simulink model "SPEED_CALCULATOIN"  (R2024b)
settings: Solver=FixedStepDiscrete  StartTime=0.0  StopTime=10.0  FixedStep=0.001  RelTol=1e-3
undefined symbols (not defined in the file): CONST_10000_u32, CONST_ONE_u8, DEFAULT_MAX_SPD_LIM_u16, DEFAULT_PAS_SPD_U16, DEFAULT_SPD_LIM_U16, ECO_MODE_SPD_LIM_u16, FITNESS_MODE_U8, MAX_SPD_VALUE_U16, MIN_SPD_VALUE_U16, PAS_FIVE_SPD_THSD_U16, PAS_FOUR_SPD_THSD_U16, PAS_ONE_SPD_THSD_U16, PAS_THREE_SPD_THSD_U16, PAS_TWO_SPD_THSD_U16, RPM_TO_KMPH_CONST_u32, SPD_BUFFER_u16, SPD_CONV_METER_u16, THROTTLE_SPD_LIM_U16, THROTTLE_THRESHOLD_U16, URBAN_MODE_SPD_LIM_u16, WALKMODE_SPD_LIM_U16
libraries: simulink x3
settings Model: DataDictionary=MCU_FOC_MAIN_DD.sldd  Creator=415  LastModifiedBy=415
settings OptimizationCC: DefaultParameterBehavior=Inlined  UseDivisionForNetSlopeComputation=on  GainParamInheritBuiltInType=on  UseFloatMulNetSlope=on  UseSpecifiedMinMax=on  InlineInvariantSignals=on  BitwiseOrLogicalOp=Bitwise operator  PassReuseOutputArgsAs=Individual arguments  ZeroExternalMemoryAtStartup=off  ZeroInternalMemoryAtStartup=off  NoFixptDivByZeroProtection=on  EfficientFloat2IntCast=on  LifeSpan=inf  OptimizeBlockOrder=speed  DifferentSizesBufferReuse=on  EfficientTunableParamExpr=on
settings DebuggingCC: SignalInfNanChecking=error  ReadBeforeWriteMsg=EnableAllAsError  WriteAfterWriteMsg=EnableAllAsError  WriteAfterReadMsg=EnableAllAsError  CheckMatrixSingularityMsg=error  IntegerOverflowMsg=error  ParameterTunabilityLossMsg=error  UnconnectedInputMsg=error  UnconnectedOutputMsg=error  UnconnectedLineMsg=error  UniqueDataStoreMsg=error  AssertControl=DisableAll  NonBusSignalsTreatedAsBus=error  IntegerSaturationMsg=error
settings HardwareCC: ProdLongLongMode=on
settings SFSimCC: CompileTimeRecursionLimit=0  EnableRuntimeRecursion=off  MATLABDynamicMemAlloc=off
settings RTWCC: Description=Embedded Coder  SystemTargetFile=ert.tlc  GenCodeOnly=on  TemplateMakefile=ert_default_tmf  GenerateReport=on  BuildConfiguration=Faster Runs  IncludeHyperlinkInReport=on  LaunchReport=on  GenerateTraceInfo=on  GenerateTraceReport=on  GenerateTraceReportSl=on  GenerateTraceReportSf=on  GenerateTraceReportEml=on  CheckMdlBeforeBuild=Warning
settings CodeAppCC: ForceParamTrailComments=on  IgnoreCustomStorageClasses=off  OperatorAnnotations=on  SimulinkDataObjDesc=on  SFDataObjDesc=on  MATLABFcnDesc=on  InsertBlockDesc=on  StateflowObjectComments=on  MATLABSourceComments=on  EnableCustomComments=on  ReqsInCode=on
settings ERTTargetCC: TargetLangStandard=C99 (ISO)  UtilityFuncGeneration=Shared location  CombineSignalStateStructs=on  SuppressErrorStatus=on  IncludeFileDelimiter=UseQuote  SupportNonFinite=off  ParenthesesLevel=Standards  CastingMode=Standards  GenerateSharedConstants=off  ERTCustomFileTemplate=example_file_process.tlc  EnableDataOwnership=on  EnableSignedLeftShifts=off  EnableSignedRightShifts=off

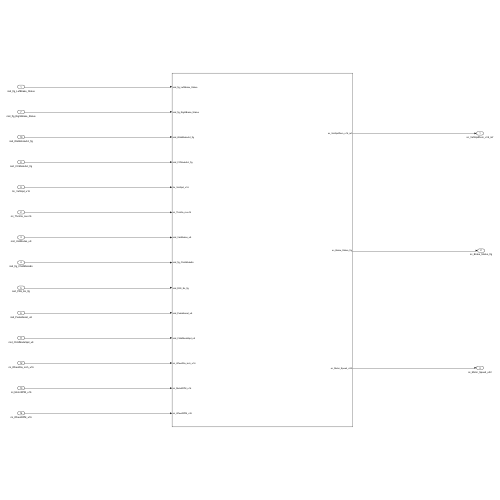
[thumbnail: Simulink's stored preview of the top-level diagram]
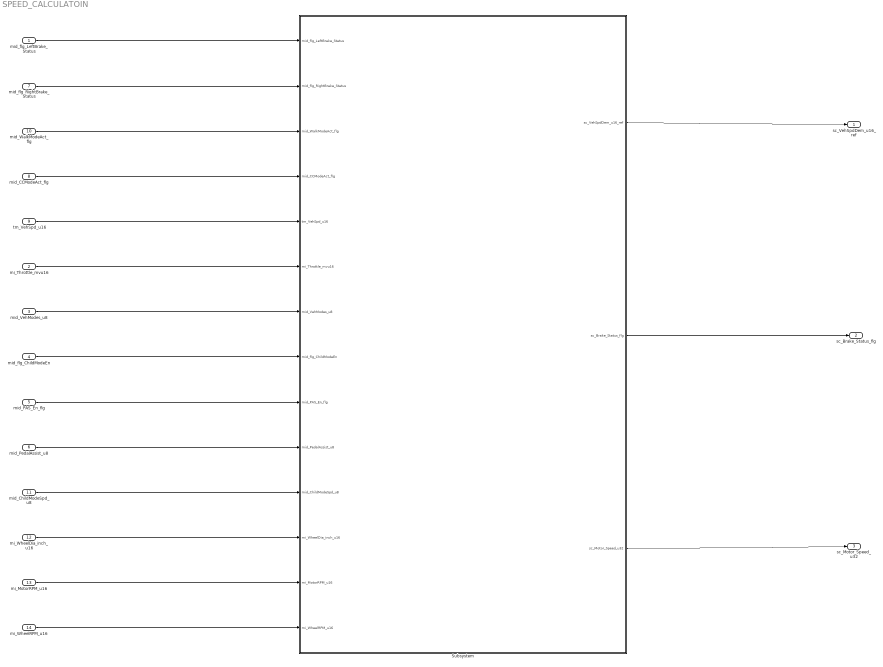
== system SPEED_CALCULATOIN ==
  mid_flg_LeftBrake_Status : Inport
  mi_Throttle_mvu16 : Inport  Port=2
  mid_VehModes_u8 : Inport  Port=3
  mid_flg_ChildModeEn : Inport  Port=4
  mid_PAS_En_flg : Inport  Port=5
  mid_PedalAssist_u8 : Inport  Port=6
  mid_flg_RightBrake_Status : Inport  Port=7
  mid_CCModeAct_flg : Inport  Port=8
  tm_VehSpd_u16 : Inport  Port=9
  mid_WalkModeAct_flg : Inport  Port=10
  mid_ChildModeSpd_u8 : Inport  Port=11
  mi_WheelDia_inch_u16 : Inport  Port=12
  mi_MotorRPM_u16 : Inport  Port=13
  mi_WheelRPM_u16 : Inport  Port=14
  Subsystem : Subsystem
  sc_VehSpdDem_u16_ref : Outport  InitialOutput=0
  sc_Brake_Status_flg : Outport  Port=2
  sc_Motor_Speed_u32 : Outport  Port=3  InitialOutput=0
  wires:
  mid_VehModes_u8/1 -> Subsystem/7(mid_VehModes_u8)
  Subsystem/2(sc_Brake_Status_flg) -> sc_Brake_Status_flg/1
  tm_VehSpd_u16/1 -> Subsystem/5(tm_VehSpd_u16)
  mid_flg_RightBrake_Status/1 -> Subsystem/2(mid_flg_RightBrake_Status)
  mid_PAS_En_flg/1 -> Subsystem/9(mid_PAS_En_flg)
  mid_flg_LeftBrake_Status/1 -> Subsystem/1(mid_flg_LeftBrake_Status)
  mid_flg_ChildModeEn/1 -> Subsystem/8(mid_flg_ChildModeEn)
  mi_Throttle_mvu16/1 -> Subsystem/6(mi_Throttle_mvu16)
  mid_CCModeAct_flg/1 -> Subsystem/4(mid_CCModeAct_flg)
  mid_WalkModeAct_flg/1 -> Subsystem/3(mid_WalkModeAct_flg)
  mid_PedalAssist_u8/1 -> Subsystem/10(mid_PedalAssist_u8)
  mid_ChildModeSpd_u8/1 -> Subsystem/11(mid_ChildModeSpd_u8)
  mi_WheelDia_inch_u16/1 -> Subsystem/12(mi_WheelDia_inch_u16)
  mi_MotorRPM_u16/1 -> Subsystem/13(mi_MotorRPM_u16)
  mi_WheelRPM_u16/1 -> Subsystem/14(mi_WheelRPM_u16)
  Subsystem/1(sc_VehSpdDem_u16_ref) -> sc_VehSpdDem_u16_ref/1
  Subsystem/3(sc_Motor_Speed_u32) -> sc_Motor_Speed_u32/1

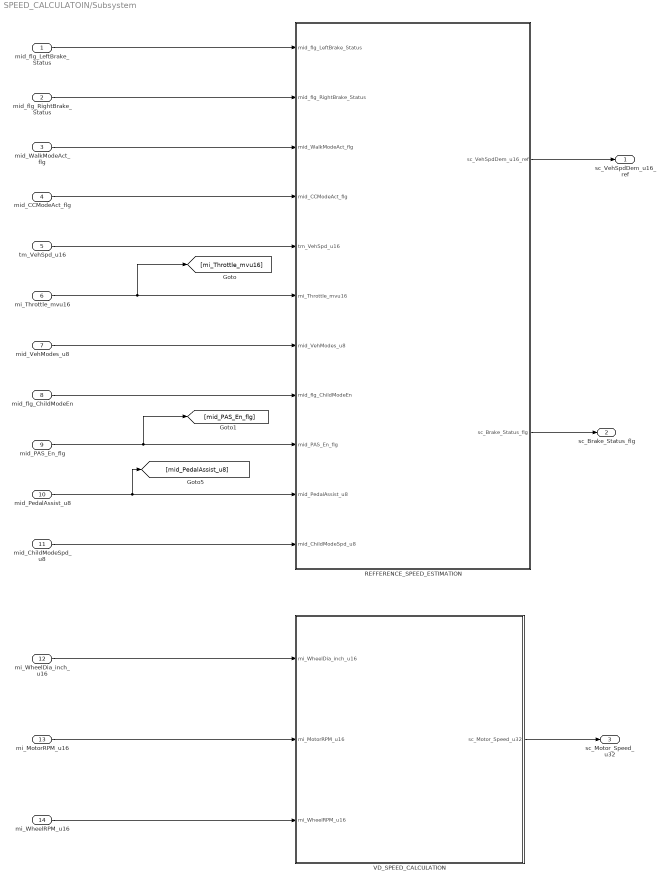
== system SPEED_CALCULATOIN/Subsystem ==
  mid_flg_LeftBrake_Status : Inport
  mid_flg_RightBrake_Status : Inport  Port=2
  mid_WalkModeAct_flg : Inport  Port=3
  mid_CCModeAct_flg : Inport  Port=4
  tm_VehSpd_u16 : Inport  Port=5
  mi_Throttle_mvu16 : Inport  Port=6
  mid_VehModes_u8 : Inport  Port=7
  mid_flg_ChildModeEn : Inport  Port=8
  mid_PAS_En_flg : Inport  Port=9
  mid_PedalAssist_u8 : Inport  Port=10
  mid_ChildModeSpd_u8 : Inport  Port=11
  mi_WheelDia_inch_u16 : Inport  Port=12
  mi_MotorRPM_u16 : Inport  Port=13
  mi_WheelRPM_u16 : Inport  Port=14
  REFFERENCE_SPEED_ESTIMATION : Subsystem
  VD_SPEED_CALCULATION : Subsystem
  sc_VehSpdDem_u16_ref : Outport
  sc_Brake_Status_flg : Outport  Port=2
  sc_Motor_Speed_u32 : Outport  Port=3
  wires:
  mid_PAS_En_flg/1 -> [mid_PAS_En_flg], REFFERENCE_SPEED_ESTIMATION/9(mid_PAS_En_flg)
  mid_PedalAssist_u8/1 -> [mid_PedalAssist_u8], REFFERENCE_SPEED_ESTIMATION/10(mid_PedalAssist_u8)
  mid_ChildModeSpd_u8/1 -> REFFERENCE_SPEED_ESTIMATION/11(mid_ChildModeSpd_u8)
  mid_VehModes_u8/1 -> REFFERENCE_SPEED_ESTIMATION/7(mid_VehModes_u8)
  mid_flg_RightBrake_Status/1 -> REFFERENCE_SPEED_ESTIMATION/2(mid_flg_RightBrake_Status)
  mid_flg_ChildModeEn/1 -> REFFERENCE_SPEED_ESTIMATION/8(mid_flg_ChildModeEn)
  mi_Throttle_mvu16/1 -> REFFERENCE_SPEED_ESTIMATION/6(mi_Throttle_mvu16), [mi_Throttle_mvu16]
  mi_WheelRPM_u16/1 -> VD_SPEED_CALCULATION/3(mi_WheelRPM_u16)
  VD_SPEED_CALCULATION/1(sc_Motor_Speed_u32) -> sc_Motor_Speed_u32/1
  REFFERENCE_SPEED_ESTIMATION/2(sc_Brake_Status_flg) -> sc_Brake_Status_flg/1
  mid_CCModeAct_flg/1 -> REFFERENCE_SPEED_ESTIMATION/4(mid_CCModeAct_flg)
  mi_WheelDia_inch_u16/1 -> VD_SPEED_CALCULATION/1(mi_WheelDia_inch_u16)
  mi_MotorRPM_u16/1 -> VD_SPEED_CALCULATION/2(mi_MotorRPM_u16)
  REFFERENCE_SPEED_ESTIMATION/1(sc_VehSpdDem_u16_ref) -> sc_VehSpdDem_u16_ref/1
  mid_WalkModeAct_flg/1 -> REFFERENCE_SPEED_ESTIMATION/3(mid_WalkModeAct_flg)
  tm_VehSpd_u16/1 -> REFFERENCE_SPEED_ESTIMATION/5(tm_VehSpd_u16)
  mid_flg_LeftBrake_Status/1 -> REFFERENCE_SPEED_ESTIMATION/1(mid_flg_LeftBrake_Status)

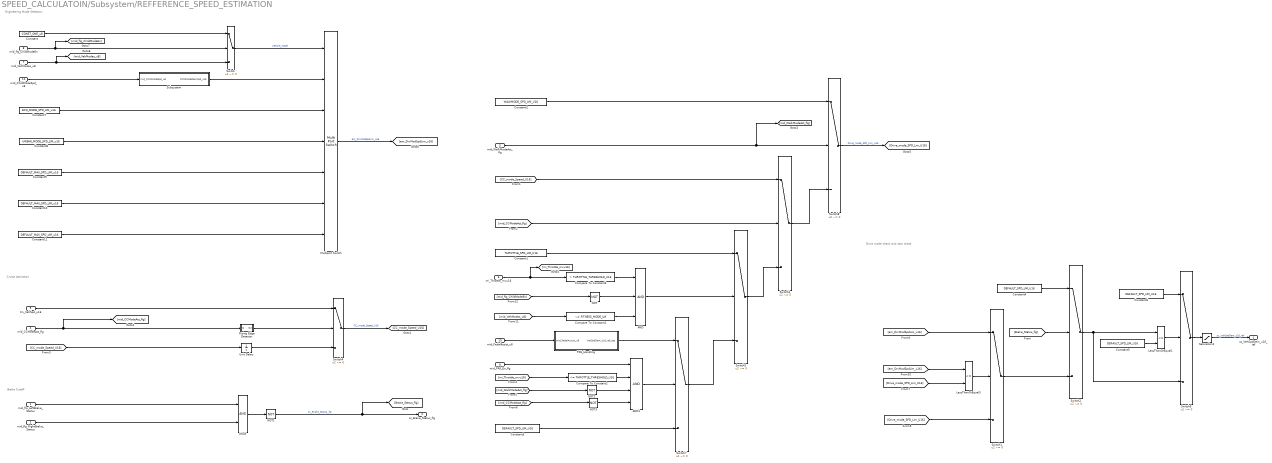
== system SPEED_CALCULATOIN/Subsystem/REFFERENCE_SPEED_ESTIMATION ==
  note: Engineering Mode Selection
  note: Drive mode check and zero check
  note: Brake Cutoff
  note: Cruise Activation
  mid_flg_LeftBrake_Status : Inport
  mid_flg_RightBrake_Status : Inport  Port=2
  mid_WalkModeAct_flg : Inport  Port=3
  mid_CCModeAct_flg : Inport  Port=4
  tm_VehSpd_u16 : Inport  Port=5
  mi_Throttle_mvu16 : Inport  Port=6
  mid_VehModes_u8 : Inport  Port=7
  mid_flg_ChildModeEn : Inport  Port=8
  mid_PAS_En_flg : Inport  Port=9
  mid_PedalAssist_u8 : Inport  Port=10
  mid_ChildModeSpd_u8 : Inport  Port=11
  AND : Logic  Inputs=3  AllPortsSameDT=off  OutDataTypeStr=boolean
  AND1 : Logic  Inputs=4  AllPortsSameDT=off  OutDataTypeStr=boolean
  AND4 : Logic  AllPortsSameDT=off  OutDataTypeStr=boolean
  Compare To Constant1 : simulink/Logic and Bit Operations/Compare To Constant  relop=~=  const=FITNESS_MODE_U8  OutDataTypeStr=boolean
  Compare To Constant2 : simulink/Logic and Bit Operations/Compare To Constant  relop=<=  const=THROTTLE_THRESHOLD_U16  OutDataTypeStr=boolean
  Compare To Constant3 : simulink/Logic and Bit Operations/Compare To Constant  relop=>  const=THROTTLE_THRESHOLD_U16  OutDataTypeStr=boolean
  Constant : Constant  Value=CONST_ONE_u8
  Constant1 : Constant  Value=THROTTLE_SPD_LIM_U16
  Constant10 : Constant  Value=DEFAULT_MAX_SPD_LIM_u16
  Constant11 : Constant  Value=DEFAULT_MAX_SPD_LIM_u16
  Constant2 : Constant  Value=WALKMODE_SPD_LIM_U16
  Constant{3..6} (4 alike) : Constant  Value=DEFAULT_SPD_LIM_U16
  Constant7 : Constant  Value=ECO_MODE_SPD_LIM_u16
  Constant8 : Constant  Value=URBAN_MODE_SPD_LIM_u16
  Constant9 : Constant  Value=DEFAULT_MAX_SPD_LIM_u16
  LessThanOrEqual1 : RelationalOperator  Operator=<=  OutDataTypeStr=boolean  RndMeth=Simplest  InputSameDT=off
  LessThanOrEqual3 : RelationalOperator  Operator=<=  OutDataTypeStr=boolean  RndMeth=Simplest  InputSameDT=off
  Multiport Switch : MultiPortSwitch  DataPortOrder=Specify indices  DataPortIndices={1,2,3,4,5,6}  DiagnosticForDefault=Warning  SaturateOnIntegerOverflow=off  InputSameDT=off
  NOT{,1..3} (4 alike) : Logic  Operator=NOT  IconShape=distinctive  AllPortsSameDT=off  OutDataTypeStr=boolean
  PAS_Handling : Subsystem
  Rising Edge Detector : Subsystem
  Saturation2 : Saturate  UpperLimit=MAX_SPD_VALUE_U16  LowerLimit=MIN_SPD_VALUE_U16
  Subsystem : Subsystem
  Switch{,1..8} (9 alike) : Switch  Criteria=u2 ~= 0  SaturateOnIntegerOverflow=off  InputSameDT=off
  Unit Delay : UnitDelay  SampleTime=-1  HasFrameUpgradeWarning=on
  sc_VehSpdDem_u16_ref : Outport  InitialOutput=0
  sc_Brake_Status_flg : Outport  Port=2
  wires:
  Saturation2/1 -> sc_VehSpdDem_u16_ref/1  "sc_VehSpdDem_u16_ref"
  Switch2/1 -> Switch6/3, LessThanOrEqual1/1
  Constant5/1 -> LessThanOrEqual1/2
  LessThanOrEqual1/1 -> Switch6/2
  Constant6/1 -> Switch6/1
  mid_flg_RightBrake_Status/1 -> AND4/2
  Constant4/1 -> Switch2/1
  Switch1/1 -> Switch2/3
  NOT1/1 -> sc_Brake_Status_flg/1, [Brake_Status_flg]  "sc_Brake_Status_flg"
  mid_flg_LeftBrake_Status/1 -> AND4/1
  AND4/1 -> NOT1/1
  Switch6/1 -> Saturation2/1
  [Brake_Status_flg] -> Switch2/2
  [em_DrvModSpdLim_u16] -> LessThanOrEqual3/1
  [Drive_mode_SPD_Lim_U16] -> LessThanOrEqual3/2
  mid_WalkModeAct_flg/1 -> [mid_WalkModeAct_flg], Switch8/2
  Constant2/1 -> Switch8/1
  Switch3/1 -> Switch8/3
  mid_CCModeAct_flg/1 -> [mid_CCModeAct_flg], Rising Edge Detector/1(Ip)
  tm_VehSpd_u16/1 -> Switch4/1
  Rising Edge Detector/1(Op) -> Switch4/2
  Switch4/1 -> [CC_mode_Speed_U16]  "CC_mode_Speed_U16"
  Unit Delay/1 -> Switch4/3
  [mid_CCModeAct_flg] -> Switch3/2
  [CC_mode_Speed_U16] -> Switch3/1
  [CC_mode_Speed_U16] -> Unit Delay/1
  Switch5/1 -> Switch3/3
  AND/1 -> Switch5/2
  Compare To Constant3/1 -> AND/1
  Compare To Constant1/1 -> AND/3
  mid_VehModes_u8/1 -> [mid_VehModes_u8], Switch/3
  Constant1/1 -> Switch5/1
  Switch7/1 -> Switch5/3
  PAS_Handling/1(VehSpdDem_u16_ref_pas) -> Switch7/1
  mid_PedalAssist_u8/1 -> PAS_Handling/1(mid_PedalAssist_u8)
  mid_PAS_En_flg/1 -> AND1/1
  Constant3/1 -> Switch7/3
  AND1/1 -> Switch7/2
  [mid_WalkModeAct_flg] -> NOT2/1
  [mid_CCModeAct_flg] -> NOT3/1
  NOT2/1 -> AND1/3
  NOT3/1 -> AND1/4
  Compare To Constant2/1 -> AND1/2
  [mi_Throttle_mvu16] -> Compare To Constant2/1
  LessThanOrEqual3/1 -> Switch1/2
  Switch8/1 -> [Drive_mode_SPD_Lim_U16]  "Drive_mode_SPD_Lim_U16"
  [em_DrvModSpdLim_u16] -> Switch1/1
  [Drive_mode_SPD_Lim_U16] -> Switch1/3
  NOT/1 -> AND/2
  mid_flg_ChildModeEn/1 -> [mid_flg_ChildModeEn], Switch/2
  Constant/1 -> Switch/1
  mi_Throttle_mvu16/1 -> [mi_Throttle_mvu16], Compare To Constant3/1
  [mid_flg_ChildModeEn] -> NOT/1
  [mid_VehModes_u8] -> Compare To Constant1/1
  Switch/1 -> Multiport Switch/1  "Vehicle_Mode"
  mid_ChildModeSpd_u8/1 -> Subsystem/1(mid_ChildModeSpd_u8)
  Subsystem/1(ChildModeDemSpd_u16) -> Multiport Switch/2
  Constant7/1 -> Multiport Switch/3
  Constant8/1 -> Multiport Switch/4
  Constant9/1 -> Multiport Switch/5
  Constant10/1 -> Multiport Switch/6
  Constant11/1 -> Multiport Switch/7
  Multiport Switch/1 -> [em_DrvModSpdLim_u16]  "em_DrvModSpdLim_u16"

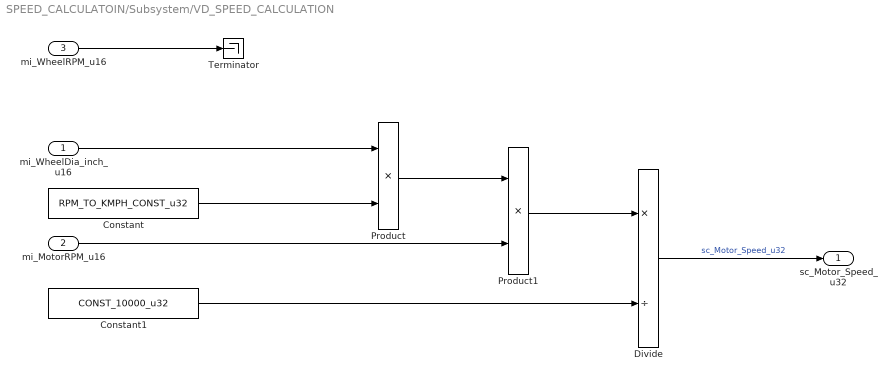
== system SPEED_CALCULATOIN/Subsystem/VD_SPEED_CALCULATION ==
  mi_WheelDia_inch_u16 : Inport
  mi_MotorRPM_u16 : Inport  Port=2
  mi_WheelRPM_u16 : Inport  Port=3
  Constant : Constant  Value=RPM_TO_KMPH_CONST_u32
  Constant1 : Constant  Value=CONST_10000_u32
  Divide : Product  Inputs=*/  OutDataTypeStr=Inherit: Inherit via back propagation
  Product : Product  OutDataTypeStr=Inherit: Inherit via back propagation
  Product1 : Product  OutDataTypeStr=Inherit: Inherit via back propagation
  Terminator : Terminator
  sc_Motor_Speed_u32 : Outport
  wires:
  Divide/1 -> sc_Motor_Speed_u32/1  "sc_Motor_Speed_u32"
  Constant1/1 -> Divide/2
  Product1/1 -> Divide/1
  mi_WheelRPM_u16/1 -> Terminator/1
  mi_MotorRPM_u16/1 -> Product1/2
  Product/1 -> Product1/1
  Constant/1 -> Product/2
  mi_WheelDia_inch_u16/1 -> Product/1

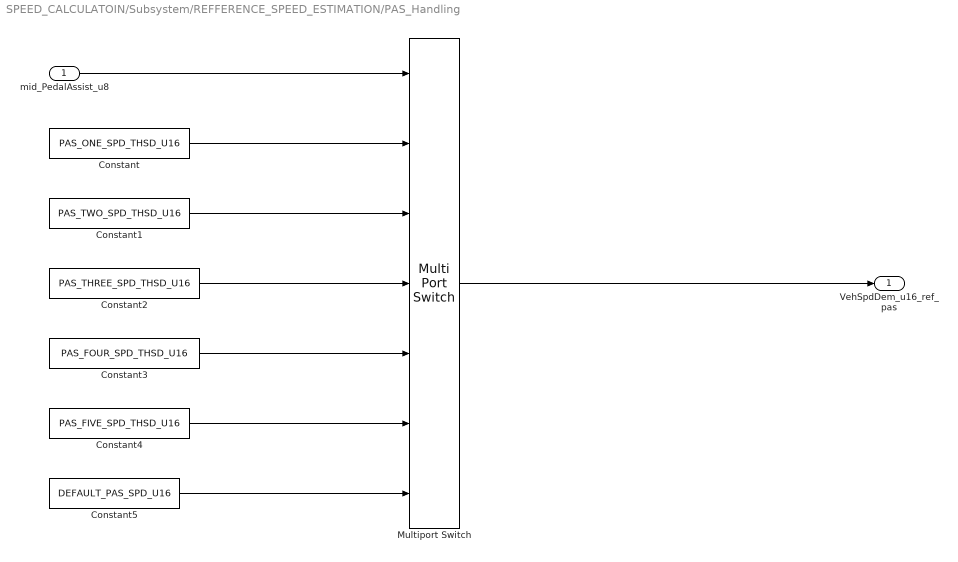
== system SPEED_CALCULATOIN/Subsystem/REFFERENCE_SPEED_ESTIMATION/PAS_Handling ==
  mid_PedalAssist_u8 : Inport
  Constant : Constant  Value=PAS_ONE_SPD_THSD_U16
  Constant1 : Constant  Value=PAS_TWO_SPD_THSD_U16
  Constant2 : Constant  Value=PAS_THREE_SPD_THSD_U16
  Constant3 : Constant  Value=PAS_FOUR_SPD_THSD_U16
  Constant4 : Constant  Value=PAS_FIVE_SPD_THSD_U16
  Constant5 : Constant  Value=DEFAULT_PAS_SPD_U16
  Multiport Switch : MultiPortSwitch  DataPortOrder=Specify indices  DataPortIndices={1,2,3,4,5}  DataPortForDefault=Additional data port  DiagnosticForDefault=None  SaturateOnIntegerOverflow=off  InputSameDT=off
  VehSpdDem_u16_ref_pas : Outport
  wires:
  mid_PedalAssist_u8/1 -> Multiport Switch/1
  Constant/1 -> Multiport Switch/2
  Constant1/1 -> Multiport Switch/3
  Constant2/1 -> Multiport Switch/4
  Constant3/1 -> Multiport Switch/5
  Constant4/1 -> Multiport Switch/6
  Constant5/1 -> Multiport Switch/7
  Multiport Switch/1 -> VehSpdDem_u16_ref_pas/1

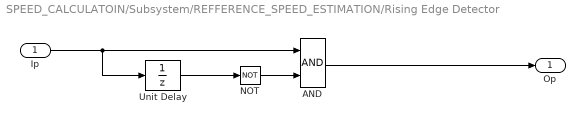
== system SPEED_CALCULATOIN/Subsystem/REFFERENCE_SPEED_ESTIMATION/Rising Edge Detector ==
  Ip : Inport
  AND : Logic  AllPortsSameDT=off  OutDataTypeStr=boolean
  NOT : Logic  Operator=NOT  IconShape=distinctive  AllPortsSameDT=off  OutDataTypeStr=boolean
  Unit Delay : UnitDelay  SampleTime=-1  HasFrameUpgradeWarning=on
  Op : Outport
  wires:
  Ip/1 -> Unit Delay/1, AND/1
  AND/1 -> Op/1
  NOT/1 -> AND/2
  Unit Delay/1 -> NOT/1

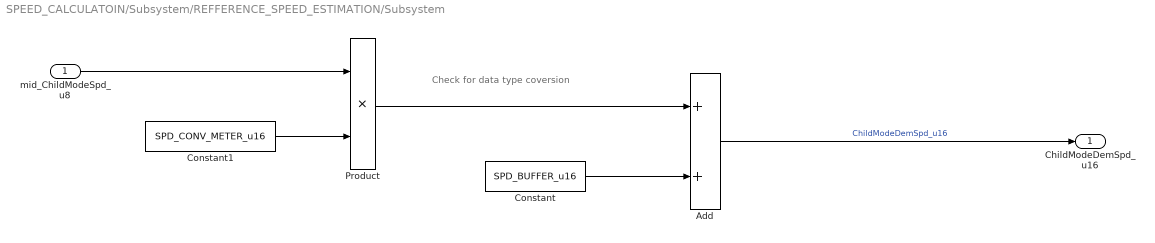
== system SPEED_CALCULATOIN/Subsystem/REFFERENCE_SPEED_ESTIMATION/Subsystem ==
  note: Check for data type coversion
  mid_ChildModeSpd_u8 : Inport
  Add : Sum
  Constant : Constant  Value=SPD_BUFFER_u16
  Constant1 : Constant  Value=SPD_CONV_METER_u16
  Product : Product
  ChildModeDemSpd_u16 : Outport
  wires:
  Constant/1 -> Add/2
  Product/1 -> Add/1
  Add/1 -> ChildModeDemSpd_u16/1  "ChildModeDemSpd_u16"
  Constant1/1 -> Product/2
  mid_ChildModeSpd_u8/1 -> Product/1
